simulink model "dae"  (R2021a)
settings: Solver=VariableStepAuto  StartTime=0.0  StopTime=20.0  RelTol=1e-3
settings Model: Creator=Suman  LastModifiedBy=Suman

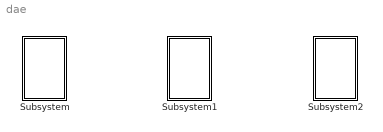
== system dae ==
  Subsystem : Subsystem
  Subsystem1 : Subsystem
  Subsystem2 : Subsystem

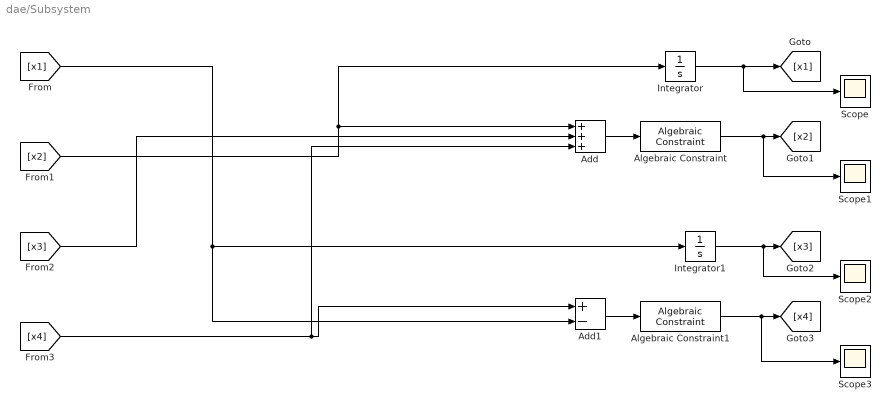
== system dae/Subsystem ==
  Add : Sum  Inputs=+++
  Add1 : Sum  Inputs=+-
  Algebraic Constraint : AlgebraicConstraint  InitialGuess=9
  Algebraic Constraint1 : AlgebraicConstraint  InitialGuess=3
  Integrator : Integrator  InitialCondition=10
  Integrator1 : Integrator  InitialCondition=2
  Scope{,1..3} (4 alike) : Scope
  wires:
  Integrator1/1 -> Scope2/1, [x3]
  Algebraic Constraint1/1 -> Scope3/1, [x4]
  [x2] -> Add/1, Integrator/1
  [x4] -> Add/3, Add1/1
  Integrator/1 -> Scope/1, [x1]
  Add/1 -> Algebraic Constraint/1
  [x1] -> Add1/2, Integrator1/1
  Algebraic Constraint/1 -> Scope1/1, [x2]
  Add1/1 -> Algebraic Constraint1/1
  [x3] -> Add/2

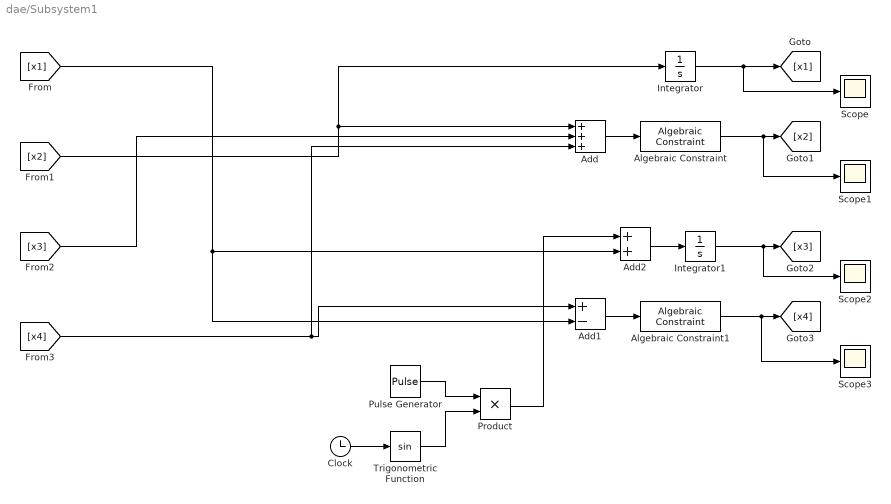
== system dae/Subsystem1 ==
  Add : Sum  Inputs=+++
  Add1 : Sum  Inputs=+-
  Add2 : Sum
  Algebraic Constraint : AlgebraicConstraint  InitialGuess=-10
  Algebraic Constraint1 : AlgebraicConstraint
  Clock : Clock
  Integrator : Integrator  InitialCondition=10
  Integrator1 : Integrator  InitialCondition=2
  Product : Product
  Pulse Generator : DiscretePulseGenerator  PulseType=Time based  Period=20  PulseWidth=50  PhaseDelay=3
  Scope{,1..3} (4 alike) : Scope
  Trigonometric Function : Trigonometry
  wires:
  [x3] -> Add/2
  Add1/1 -> Algebraic Constraint1/1
  Algebraic Constraint/1 -> [x2], Scope1/1
  [x1] -> Add2/2, Add1/2
  Add/1 -> Algebraic Constraint/1
  Integrator/1 -> [x1], Scope/1
  [x4] -> Add1/1, Add/3
  [x2] -> Integrator/1, Add/1
  Algebraic Constraint1/1 -> [x4], Scope3/1
  Integrator1/1 -> [x3], Scope2/1
  Add2/1 -> Integrator1/1
  Pulse Generator/1 -> Product/1
  Trigonometric Function/1 -> Product/2
  Product/1 -> Add2/1
  Clock/1 -> Trigonometric Function/1

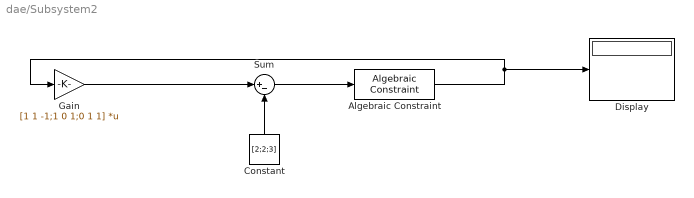
== system dae/Subsystem2 ==
  Algebraic Constraint : AlgebraicConstraint
  Constant : Constant  Value=[2;2;3]
  Display : Display
  Gain : Gain  Gain=[1 1 -1;1 0 1;0 1 1]  Multiplication=Matrix(K*u) (u vector)
  Sum : Sum  Inputs=|+-
  wires:
  Gain/1 -> Sum/1
  Algebraic Constraint/1 -> Display/1, Gain/1
  Constant/1 -> Sum/2
  Sum/1 -> Algebraic Constraint/1
